simulink model "Four_QAM_Modulation"  (R2024a)
settings: Solver=VariableStepAuto  StartTime=0.0  StopTime=10.0  RelTol=1e-3
libraries: simulink x1, commrandsrc3 x1
settings Model: Creator=alice  LastModifiedBy=alice

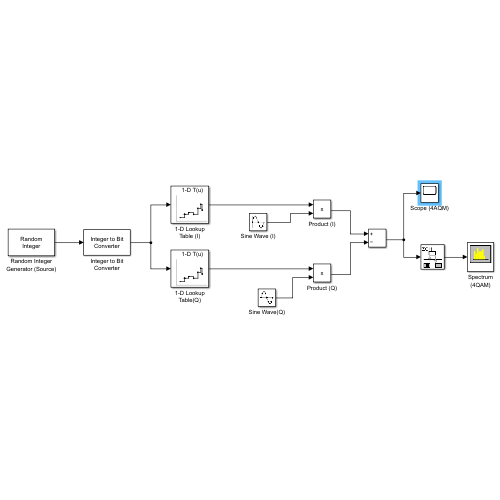
[thumbnail: Simulink's stored preview of the top-level diagram]
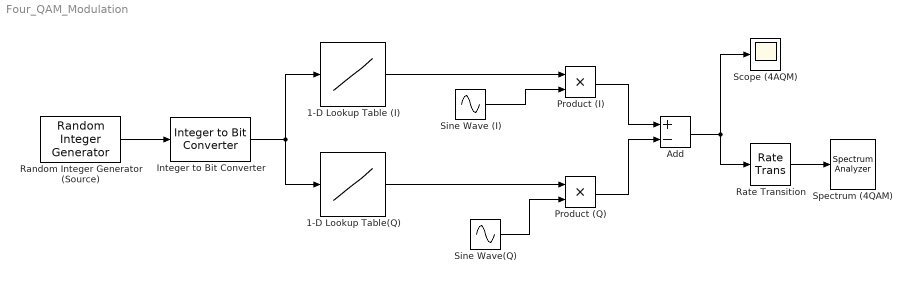
== system Four_QAM_Modulation ==
  1-D Lookup Table (I) : Lookup_n-D  NumberOfTableDimensions=1  LookupTableObject=''  BreakpointsForDimension1=[0,1]  BreakpointsForDimension1FirstPoint=10  BreakpointsForDimension2FirstPoint=10  BreakpointsForDimension1Spacing=12  BreakpointsForDimension2Spacing=12  IndexSearchMethod=Evenly spaced points  Table=[-sqrt(0.5), sqrt(0.5)]  InterpMethod=Flat  DiagnosticForOutOfRangeInput=Error  InternalRulePriority=Speed  RndMeth=Simplest
  1-D Lookup Table(Q) : Lookup_n-D  NumberOfTableDimensions=1  LookupTableObject=''  BreakpointsForDimension1=[0,1]  BreakpointsForDimension1FirstPoint=10  BreakpointsForDimension2FirstPoint=10  BreakpointsForDimension1Spacing=12  BreakpointsForDimension2Spacing=12  IndexSearchMethod=Evenly spaced points  Table=[-sqrt(0.5), sqrt(0.5)]  InterpMethod=Flat  DiagnosticForOutOfRangeInput=Error  InternalRulePriority=Speed  RndMeth=Simplest
  Add : Sum  Inputs=+-
  Integer to Bit Converter : simulink/Logic and Bit Operations/Integer to Bit Converter  nbits=2  signedInputValues=Unsigned  bitOrder=MSB first  outDtype=Inherit via internal rule
  Product (I) : Product
  Product (Q) : Product
  Random Integer Generator (Source) : commrandsrc3/Random Integer Generator  SetSize=4  SeedSource=Parameter  Seed=0  SampleTime=1e-3  SamplesPerFrame=1  OutputDataType=double  SimulateUsing=Interpreted execution
  Rate Transition : RateTransition  OutPortSampleTime=0.5e-4
  Scope (4AQM) : Scope
  Sine Wave (I) : Sin  SineType=Sample based  Samples=5000  SampleTime=1e-7  Offset=1250
  Sine Wave(Q) : Sin  SineType=Sample based  Samples=5000  SampleTime=1e-7
  Spectrum (4QAM) : SpectrumAnalyzer  WindowPosition=[1.000000,49.000000,1280.000000,729.000000,]  ScopeFrameLocation=window  YLimits=[-49.61393348,16.36843491]  SelectedToolstripTab=spectrumAnalyzerToolstrip.channelMeasurementsTab
  wires:
  Random Integer Generator (Source)/1 -> Integer to Bit Converter/1
  Integer to Bit Converter/1 -> 1-D Lookup Table(Q)/1, 1-D Lookup Table (I)/1
  1-D Lookup Table (I)/1 -> Product (I)/1
  Sine Wave (I)/1 -> Product (I)/2
  Product (I)/1 -> Add/1
  Product (Q)/1 -> Add/2
  1-D Lookup Table(Q)/1 -> Product (Q)/1
  Sine Wave(Q)/1 -> Product (Q)/2
  Add/1 -> Rate Transition/1, Scope (4AQM)/1
  Rate Transition/1 -> Spectrum (4QAM)/1
